simulink model "PitchVelocityControllers"  (R2021a)
settings: Solver=VariableStepAuto  StartTime=0.0  StopTime=500  RelTol=1e-3
undefined symbols (not defined in the file): A_long, B_long, C_long, D_long, servo, ThetaController_KD, ThetaController_KI, ThetaController_KP, UController_KD, UController_KI, UController_KP, UController_PD, UController_ZD, X0
libraries: simulink_extras x4, cstblocks x3
settings Model: Creator=User01  LastModifiedBy=User01

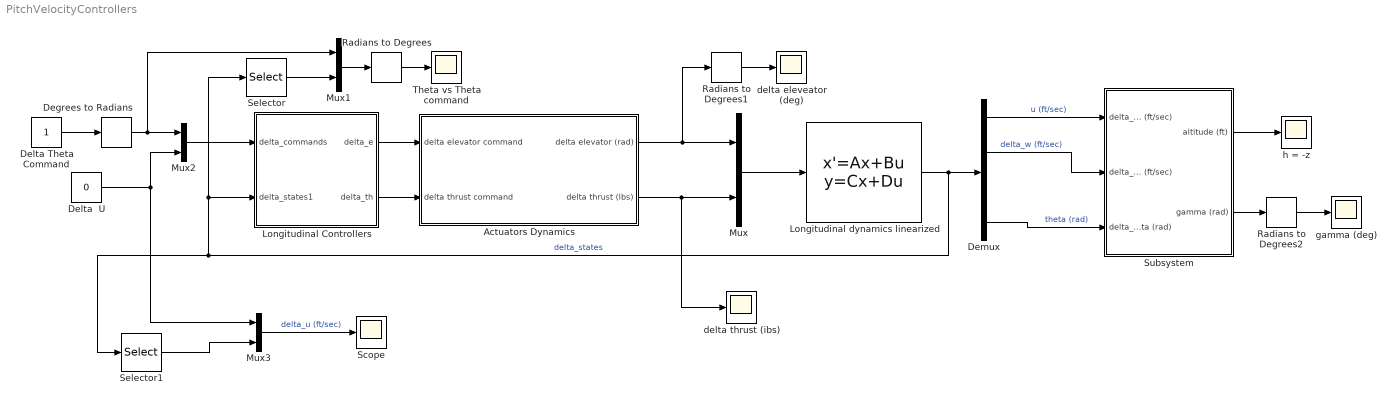
== system PitchVelocityControllers ==
  Actuators Dynamics : Subsystem
  Degrees to Radians : simulink_extras/Transformations/Degrees to Radians
  Delta  U : Constant  Value=0
  Delta Theta Command : Constant
  Demux : Demux
  Longitudinal Controllers : Subsystem
  Longitudinal dynamics linearized : StateSpace  A=A_long  B=B_long  C=C_long  D=D_long  InitialCondition=0
  Mux{,1..3} (4 alike) : Mux  Inputs=2
  Radians to Degrees : simulink_extras/Transformations/Radians to Degrees
  Radians to Degrees1 : simulink_extras/Transformations/Radians to Degrees
  Radians to Degrees2 : simulink_extras/Transformations/Radians to Degrees
  Scope : Scope
  Selector : Selector  InputPortWidth=4  IndexOptions=Index vector (dialog)  Indices=4  OutputSizes=1
  Selector1 : Selector  InputPortWidth=4  IndexOptions=Index vector (dialog)  Indices=1  OutputSizes=1
  Subsystem : Subsystem
  Theta vs Theta command : Scope
  delta eleveator (deg) : Scope
  delta thrust (ibs) : Scope
  gamma (deg) : Scope
  h = -z : Scope
  wires:
  Radians to Degrees1/1 -> delta eleveator (deg)/1
  Mux/1 -> Longitudinal dynamics linearized/1
  Delta Theta Command/1 -> Degrees to Radians/1
  Delta  U/1 -> Mux2/2, Mux3/1
  Radians to Degrees2/1 -> gamma (deg)/1
  Radians to Degrees/1 -> Theta vs Theta command/1
  Degrees to Radians/1 -> Mux2/1, Mux1/1
  Longitudinal dynamics linearized/1 -> Selector1/1, Selector/1, Longitudinal Controllers/2(delta_states1), Demux/1  "delta_states"
  Mux1/1 -> Radians to Degrees/1
  Subsystem/1(altitude (ft)) -> h = -z/1
  Subsystem/2(gamma (rad)) -> Radians to Degrees2/1
  Mux2/1 -> Longitudinal Controllers/1(delta_commands)
  Selector/1 -> Mux1/2
  Actuators Dynamics/1(delta elevator (rad)) -> Radians to Degrees1/1, Mux/1
  Longitudinal Controllers/1(delta_e) -> Actuators Dynamics/1(delta elevator command)
  Longitudinal Controllers/2(delta_th) -> Actuators Dynamics/2(delta thrust command)
  Actuators Dynamics/2(delta thrust (lbs)) -> delta thrust (ibs)/1, Mux/2
  Demux/2 -> Subsystem/2(delta_w (ft/sec))  "delta_w (ft/sec)"
  Demux/4 -> Subsystem/3(delta_theta (rad))  "theta (rad)"
  Demux/1 -> Subsystem/1(delta_u (ft/sec))  "u (ft/sec)"
  Selector1/1 -> Mux3/2
  Mux3/1 -> Scope/1  "delta_u (ft/sec)"

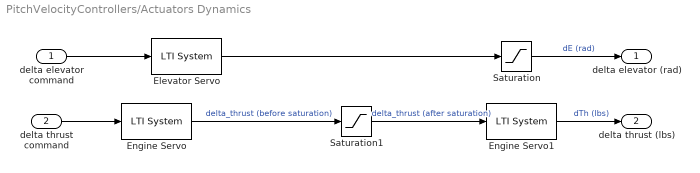
== system PitchVelocityControllers/Actuators Dynamics ==
  delta elevator command : Inport
  delta thrust command : Inport  Port=2
  Elevator Servo : cstblocks/LTI System  sys=-servo  IC=[]
  Engine Servo : cstblocks/LTI System  sys=servo  IC=[]
  Engine Servo1 : cstblocks/LTI System  sys=engine_timelag  IC=[]
  Saturation : Saturate  UpperLimit=25*pi/180  LowerLimit=-25*pi/180
  Saturation1 : Saturate  UpperLimit=47000  LowerLimit=-141000
  delta elevator (rad) : Outport
  delta thrust (lbs) : Outport  Port=2
  wires:
  Saturation/1 -> delta elevator (rad)/1  "dE (rad)"
  delta thrust command/1 -> Engine Servo/1
  Elevator Servo/1 -> Saturation/1
  Saturation1/1 -> Engine Servo1/1  "delta_thrust (after saturation)"
  Engine Servo/1 -> Saturation1/1  "delta_thrust (before saturation)"
  Engine Servo1/1 -> delta thrust (lbs)/1  "dTh (lbs)"
  delta elevator command/1 -> Elevator Servo/1

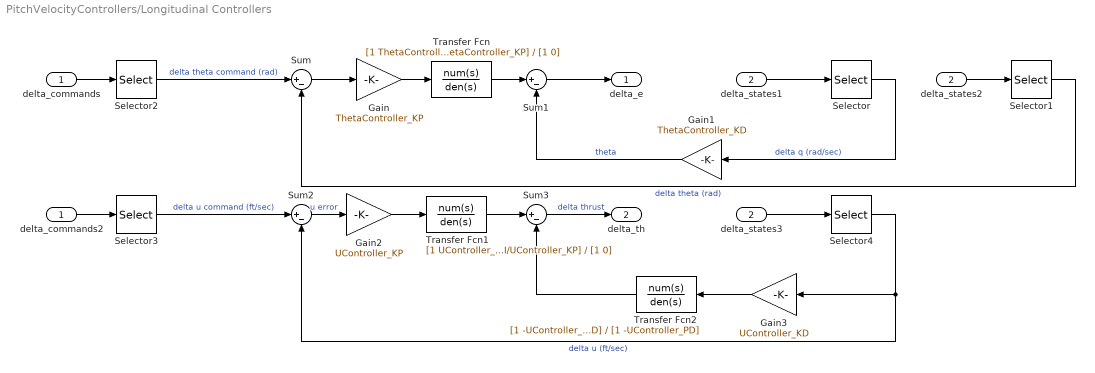
== system PitchVelocityControllers/Longitudinal Controllers ==
  delta_commands : Inport
  delta_states1 : Inport  Port=2
  Gain : Gain  Gain=ThetaController_KP
  Gain1 : Gain  Gain=ThetaController_KD
  Gain2 : Gain  Gain=UController_KP
  Gain3 : Gain  Gain=UController_KD
  Selector : Selector  InputPortWidth=4  IndexOptions=Index vector (dialog)  Indices=3  OutputSizes=1
  Selector1 : Selector  InputPortWidth=4  IndexOptions=Index vector (dialog)  Indices=4  OutputSizes=1
  Selector2 : Selector  InputPortWidth=2  IndexOptions=Index vector (dialog)  Indices=1  OutputSizes=1
  Selector3 : Selector  InputPortWidth=2  IndexOptions=Index vector (dialog)  Indices=2  OutputSizes=1
  Selector4 : Selector  InputPortWidth=4  IndexOptions=Index vector (dialog)  Indices=1  OutputSizes=1
  Sum{,1..3} (4 alike) : Sum  Inputs=|+-
  Transfer Fcn : TransferFcn  Numerator=[1 ThetaController_KI/ThetaController_KP]  Denominator=[1 0]
  Transfer Fcn1 : TransferFcn  Numerator=[1 UController_KI/UController_KP]  Denominator=[1 0]
  Transfer Fcn2 : TransferFcn  Numerator=[1 -UController_ZD]  Denominator=[1 -UController_PD]
  delta_commands2 : InportShadow
  delta_states2 : InportShadow  Port=2
  delta_states3 : InportShadow  Port=2
  delta_e : Outport
  delta_th : Outport  Port=2
  wires:
  Sum1/1 -> delta_e/1
  Transfer Fcn/1 -> Sum1/1
  Gain/1 -> Transfer Fcn/1
  Gain1/1 -> Sum1/2  "theta"
  Sum/1 -> Gain/1
  delta_commands/1 -> Selector2/1
  Selector2/1 -> Sum/1  "delta theta command (rad)"
  delta_states1/1 -> Selector/1
  Selector/1 -> Gain1/1  "delta q (rad/sec)"
  delta_states2/1 -> Selector1/1
  Selector1/1 -> Sum/2  "delta theta (rad)"
  delta_commands2/1 -> Selector3/1
  delta_states3/1 -> Selector4/1
  Selector3/1 -> Sum2/1  "delta u command (ft/sec)"
  Selector4/1 -> Gain3/1, Sum2/2  "delta u (ft/sec)"
  Transfer Fcn1/1 -> Sum3/1
  Sum2/1 -> Gain2/1  "u error"
  Sum3/1 -> delta_th/1  "delta thrust"
  Transfer Fcn2/1 -> Sum3/2
  Gain2/1 -> Transfer Fcn1/1
  Gain3/1 -> Transfer Fcn2/1

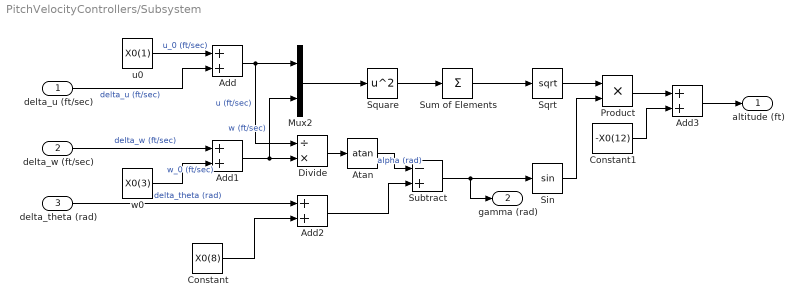
== system PitchVelocityControllers/Subsystem ==
  delta_u (ft/sec) : Inport
  delta_w (ft/sec) : Inport  Port=2
  delta_theta (rad) : Inport  Port=3
  Add{,1..3} (4 alike) : Sum
  Atan : Trigonometry  Operator=atan
  Constant : Constant  Value=X0(8)
  Constant1 : Constant  Value=-X0(12)
  Divide : Product  Inputs=/*
  Mux2 : Mux  Inputs=2
  Product : Product
  Sin : Trigonometry
  Sqrt : Sqrt  SaturateOnIntegerOverflow=on
  Square : Math  Operator=square  SaturateOnIntegerOverflow=on
  Subtract : Sum  Inputs=-+
  Sum of Elements : Sum  Inputs=+
  u0 : Constant  Value=X0(1)
  w0 : Constant  Value=X0(3)
  altitude (ft) : Outport
  gamma (rad) : Outport  Port=2
  wires:
  Subtract/1 -> gamma (rad)/1, Sin/1
  delta_u (ft/sec)/1 -> Add/2  "delta_u (ft/sec)"
  Add/1 -> Divide/1, Mux2/1  "u (ft/sec)"
  delta_w (ft/sec)/1 -> Add1/1  "delta_w (ft/sec)"
  Constant/1 -> Add2/2
  Sin/1 -> Product/2
  delta_theta (rad)/1 -> Add2/1  "delta_theta (rad)"
  Product/1 -> Add3/1
  u0/1 -> Add/1  "u_0 (ft/sec)"
  w0/1 -> Add1/2  "w_0 (ft/sec)"
  Sum of Elements/1 -> Sqrt/1
  Mux2/1 -> Square/1
  Square/1 -> Sum of Elements/1
  Add2/1 -> Subtract/2
  Atan/1 -> Subtract/1  "alpha (rad)"
  Constant1/1 -> Add3/2
  Add3/1 -> altitude (ft)/1
  Sqrt/1 -> Product/1
  Add1/1 -> Mux2/2, Divide/2  "w (ft/sec)"
  Divide/1 -> Atan/1
